simulink model "success"  (R2018a)
settings: Solver=ode4  StartTime=0.0  StopTime=50  FixedStep=0.005  RelTol=1e-3
settings Model: Creator=Vishesh  LastModifiedBy=Vishesh

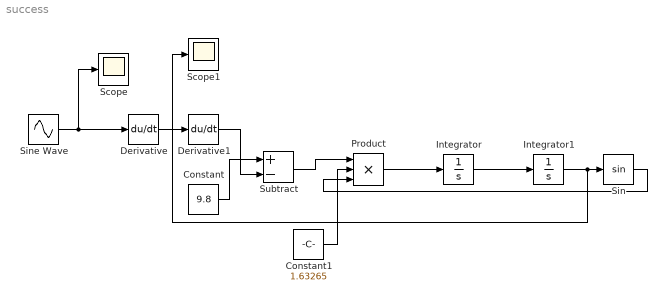
== system success ==
  Constant : Constant  Value=9.8
  Constant1 : Constant  Value=1.63265
  Derivative : Derivative
  Derivative1 : Derivative
  Integrator : Integrator
  Integrator1 : Integrator  InitialCondition=0.017
  Product : Product  Inputs=3
  Scope : Scope
  Scope1 : Scope
  Sin : Trigonometry
  Sine Wave : Sin  Amplitude=0.25  Frequency=260  Phase=1.57  SampleTime=0.005
  Subtract : Sum  Inputs=+-
  wires:
  Sine Wave/1 -> Derivative/1, Scope/1
  Derivative/1 -> Derivative1/1
  Constant1/1 -> Product/2
  Product/1 -> Integrator/1
  Integrator/1 -> Integrator1/1
  Integrator1/1 -> Scope1/1, Sin/1
  Sin/1 -> Product/3
  Derivative1/1 -> Subtract/2
  Constant/1 -> Subtract/1
  Subtract/1 -> Product/1
